simulink model "SimulinkPinson"  (R2019b)
settings: Solver=VariableStepAuto  StartTime=0.0  StopTime=6031  RelTol=1e-3
libraries: sharedTrackingLibrary x1, simulink x1
settings Model: Creator=pieterpinson  LastModifiedBy=pieterpinson

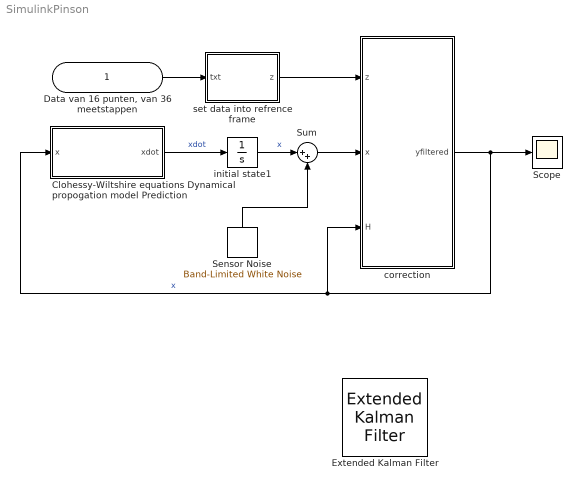
== system SimulinkPinson ==
  "Data van 16 punten, van 36 meetstappen" : Inport
  Clohessy-Wiltshire equations Dynamical propogation model Prediction : MATLAB Function  TreatAsAtomicUnit=on
  Extended Kalman Filter : sharedTrackingLibrary/Extended Kalman Filter  StateTransitionFcn=myStateTransitionFcn  HasStateTransitionJacobianFcn=off  HasAdditiveProcessNoise=Additive  ProcessNoise=1  HasTimeVaryingProcessNoise=off  HasStateTransitionFcnExtraArgument=0  InitialState=0  InitialStateCovariance=1  MeasurementFcn1=myMeasurementFcn  HasMeasurementJacobianFcn1=off  HasMeasurementEnablePort1=off  HasAdditiveMeasurementNoise1=Additive  MeasurementNoise1=1  HasTimeVaryingMeasurementNoise1=off  HasMeasurementFcnExtraArgument1=0  MeasurementFcn2=myMeasurementFcn  HasMeasurementJacobianFcn2=off  HasMeasurementEnablePort2=off  HasAdditiveMeasurementNoise2=Additive  MeasurementNoise2=1  HasTimeVaryingMeasurementNoise2=off  HasMeasurementFcnExtraArgument2=0  MeasurementFcn3=myMeasurementFcn  HasMeasurementJacobianFcn3=off  HasMeasurementEnablePort3=off  HasAdditiveMeasurementNoise3=Additive  MeasurementNoise3=1  HasTimeVaryingMeasurementNoise3=off  HasMeasurementFcnExtraArgument3=0  MeasurementFcn4=myMeasurementFcn  HasMeasurementJacobianFcn4=off  HasMeasurementEnablePort4=off  HasAdditiveMeasurementNoise4=Additive  MeasurementNoise4=1  HasTimeVaryingMeasurementNoise4=off  HasMeasurementFcnExtraArgument4=0  MeasurementFcn5=myMeasurementFcn  HasMeasurementJacobianFcn5=off  HasMeasurementEnablePort5=off  HasAdditiveMeasurementNoise5=Additive  MeasurementNoise5=1  HasTimeVaryingMeasurementNoise5=off  HasMeasurementFcnExtraArgument5=0  EnableMultirate=off  StateTransitionFcnSampleTime=1  MeasurementFcn1SampleTime=1  MeasurementFcn2SampleTime=1  MeasurementFcn3SampleTime=1  MeasurementFcn4SampleTime=1  MeasurementFcn5SampleTime=1  UseCurrentEstimator=on  OutputStateCovariance=off  DataType=double  SampleTime=1  NumberOfMeasurements=1
      settings: SourceProductName=Automated Driving Toolbox  SourceProductBaseCode=DR
  Scope : Scope
  Sensor Noise : simulink/Sources/Band-Limited White Noise  Cov=[0.1]  Ts=0.1  seed=[23341]
  Sum : Sum  Inputs=|++
  correction : MATLAB Function  TreatAsAtomicUnit=on
  initial state1 : Integrator  InitialCondition=|
      | [-2.9671 ; 0.5236
      | ; -1.3963 ; -0.0873 ; -0.1489 ; 0.0262]
  set data into refrence frame : MATLAB Function  TreatAsAtomicUnit=on
  wires:
  "Data van 16 punten, van 36 meetstappen"/1 -> set data into refrence frame/1(txt)
  Clohessy-Wiltshire equations Dynamical propogation model Prediction/1(xdot) -> initial state1/1  "xdot"
  Sensor Noise/1 -> Sum/2
  set data into refrence frame/1(z) -> correction/1(z)
  Sum/1 -> correction/2(x)
  correction/1(yfiltered) -> Scope/1, correction/3(H), Clohessy-Wiltshire equations Dynamical propogation model Prediction/1(x)  "x"
  initial state1/1 -> Sum/1  "x"

== matlab function SimulinkPinson/set data into refrence frame ==
  data: txt input; z output
function z = measurements(txt)

    z = 239/txt;
end

== matlab function SimulinkPinson/Clohessy-Wiltshire equations Dynamical propogation model Prediction ==
  data: x input; xdot output
function xdot = SCmodel(x)

Q = 10^-6*[1 ;1 ;1];

thetadot = A*x;
omegadot = Omega*P*omega + Q;

xdot = [thetadot omegadot];

end

== matlab function SimulinkPinson/correction ==
  data: z input; x input; H input; yfiltered output
function yfiltered = Kalmanfilter(z,x,H)

    K = 0.1*[1 ; 1 ; 1];%kalman gain
    
    yfiltered = x + K*(z-H);
    
end
